simulink library "simetranss"  (R2024b)
settings: Solver=VariableStepAuto  StartTime=0.0  StopTime=10.0  RelTol=1e-3
PostLoadFcn:
  | Ts=1e-6
InitFcn:
  | Ts=1e-6
undefined symbols (not defined in the file): C, C_601, C_603, C_606, CC, Csnu, Csnubber, DiscIntNeverNeededParam, DPL, DPL1ph, FluxTable, ft2km, gcbh, h, Half, Imap2, L, L_601, L_603, L_606, Lbase, LpejoSw, Newton, R_601, R_603, R_606, Raphson, ResistanceM, Roff, Ron, RotorAngles, Rsnu, Rsnubber, Rt4, SampleTime, simetran, sps, sps_rtmsupport, StatorCurrents, T_2wind_ratio, T_Lpu, T_Lpu_pri, T_Rpu, T_Rpu_pri, T_Vpri, T_Vpri_15comp, T_Vsec, Ti, Ts_Power, Z, Zbase, Zm
libraries: fl_lib x248, ee_lib x146, nesl_utility x122, $bdroot x29, simulink x15, eeGeneralControl x2, spsStairGeneratorLib x2, artemis x1
(part 11 of 12)

== system simetranss/Passive/MATE Unbalanced LoadDEV1/RLseriesD ==
  Inductor : ee_lib/Passive/Inductor  l=L(1) H  enable_L_tol=ee.enum.toleranceApplication.none  L_tol=20  tol_distribution=ee.enum.toleranceDistribution.uniform  nSigma=4  r=0 Ohm  g=1e-9 1/Ohm  enable_operating_limits=ee.enum.enable.no  operating_limit_action=ee.enum.passive.reportOpLim.warn  max_working_current=1 A  power_rating=1 W  fault_action=simscape.enum.assert.action.none  t_fault=1 s  i_L_specify=off  i_L_priority=High  i_L=0 A  i_L_nominal_specify=off  i_L_nominal_value=1  i_L_nominal_unit=A
  Inductor1 : ee_lib/Passive/Inductor  l=L(2) H  enable_L_tol=ee.enum.toleranceApplication.none  L_tol=20  tol_distribution=ee.enum.toleranceDistribution.uniform  nSigma=4  r=0 Ohm  g=1e-9 1/Ohm  enable_operating_limits=ee.enum.enable.no  operating_limit_action=ee.enum.passive.reportOpLim.warn  max_working_current=1 A  power_rating=1 W  fault_action=simscape.enum.assert.action.none  t_fault=1 s  i_L_specify=off  i_L_priority=High  i_L=0 A  i_L_nominal_specify=off  i_L_nominal_value=1  i_L_nominal_unit=A
  Inductor2 : ee_lib/Passive/Inductor  l=L(3) H  enable_L_tol=ee.enum.toleranceApplication.none  L_tol=20  tol_distribution=ee.enum.toleranceDistribution.uniform  nSigma=4  r=0 Ohm  g=1e-9 1/Ohm  enable_operating_limits=ee.enum.enable.no  operating_limit_action=ee.enum.passive.reportOpLim.warn  max_working_current=1 A  power_rating=1 W  fault_action=simscape.enum.assert.action.none  t_fault=1 s  i_L_specify=off  i_L_priority=High  i_L=0 A  i_L_nominal_specify=off  i_L_nominal_value=1  i_L_nominal_unit=A
  Phase Splitter2 : ee_lib/Connectors & References/Phase Splitter
  Resistor : ee_lib/Passive/Resistor  R=R(1) Ohm  enable_R_tol=ee.enum.toleranceApplication.none  R_tol=5  tol_distribution=ee.enum.toleranceDistribution.uniform  nSigma=4  enable_operating_limits=ee.enum.enable.no  operating_limit_action=ee.enum.passive.reportOpLim.warn  power_rating=1 W  max_working_voltage=100 V  noise_mode=ee.enum.sources.noise.Disabled  Tdevice=25 degC  sample_time=1e-3 s  repeatability=ee.enum.ic.repeatability.notRepeatable  user_seed=0  auto_seed=1853927660  fault_action=simscape.enum.assert.action.none  t_fault=1 s  power_derating_T1=70 degC  power_derating_T2=155 degC  operating_temperature_range_vec=[-50, 150] degC  alpha=3.93e-3 1/K  Tmeas=25 degC  thermal_mass=100 J/K  temperature_specify=off  temperature_priority=High  temperature=298.15 K  temperature_nominal_specify=off  temperature_nominal_value=1  temperature_nominal_unit=K
  Resistor1 : ee_lib/Passive/Resistor  R=R(2) Ohm  enable_R_tol=ee.enum.toleranceApplication.none  R_tol=5  tol_distribution=ee.enum.toleranceDistribution.uniform  nSigma=4  enable_operating_limits=ee.enum.enable.no  operating_limit_action=ee.enum.passive.reportOpLim.warn  power_rating=1 W  max_working_voltage=100 V  noise_mode=ee.enum.sources.noise.Disabled  Tdevice=25 degC  sample_time=1e-3 s  repeatability=ee.enum.ic.repeatability.notRepeatable  user_seed=0  auto_seed=66516699  fault_action=simscape.enum.assert.action.none  t_fault=1 s  power_derating_T1=70 degC  power_derating_T2=155 degC  operating_temperature_range_vec=[-50, 150] degC  alpha=3.93e-3 1/K  Tmeas=25 degC  thermal_mass=100 J/K  temperature_specify=off  temperature_priority=High  temperature=298.15 K  temperature_nominal_specify=off  temperature_nominal_value=1  temperature_nominal_unit=K
  Resistor2 : ee_lib/Passive/Resistor  R=R(3) Ohm  enable_R_tol=ee.enum.toleranceApplication.none  R_tol=5  tol_distribution=ee.enum.toleranceDistribution.uniform  nSigma=4  enable_operating_limits=ee.enum.enable.no  operating_limit_action=ee.enum.passive.reportOpLim.warn  power_rating=1 W  max_working_voltage=100 V  noise_mode=ee.enum.sources.noise.Disabled  Tdevice=25 degC  sample_time=1e-3 s  repeatability=ee.enum.ic.repeatability.notRepeatable  user_seed=0  auto_seed=4226521513  fault_action=simscape.enum.assert.action.none  t_fault=1 s  power_derating_T1=70 degC  power_derating_T2=155 degC  operating_temperature_range_vec=[-50, 150] degC  alpha=3.93e-3 1/K  Tmeas=25 degC  thermal_mass=100 J/K  temperature_specify=off  temperature_priority=High  temperature=298.15 K  temperature_nominal_specify=off  temperature_nominal_value=1  temperature_nominal_unit=K
  Conn1 : PMIOPort  Side=Left
  connections:
  Inductor2/LConn1 -- Resistor2/RConn1
  Inductor/LConn1 -- Resistor/RConn1
  Inductor1/LConn1 -- Resistor1/RConn1
  Conn1/RConn1 -- Phase Splitter2/LConn1
  Phase Splitter2/RConn1 -- Inductor2/RConn1 -- Resistor/LConn1
  Inductor/RConn1 -- Resistor1/LConn1 -- Phase Splitter2/RConn2
  Inductor1/RConn1 -- Resistor2/LConn1 -- Phase Splitter2/RConn3

== system simetranss/Power converters/MATE_3LevelNPCinverter/Subsystem ==
  g : Inport
  Capacitor : fl_lib/Electrical/Electrical Elements/Capacitor  c=SnubberCapacitance F  r=0 Ohm  g=0 1/Ohm  i_specify=off  i_priority=None  i=0 A  i_nominal_specify=off  i_nominal_value=1  i_nominal_unit=A  v_specify=off  v_priority=None  v=0 V  v_nominal_specify=off  v_nominal_value=1  v_nominal_unit=V  vc_specify=off  vc_priority=High  vc=0 V  vc_nominal_specify=off  vc_nominal_value=1  vc_nominal_unit=V
  Resistor : fl_lib/Electrical/Electrical Elements/Resistor  R=SnubberResistance Ohm  i_specify=off  i_priority=None  i=0 A  i_nominal_specify=off  i_nominal_value=1  i_nominal_unit=A  v_specify=off  v_priority=None  v=0 V  v_nominal_specify=off  v_nominal_value=1  v_nominal_unit=V
  SPST Switch : ee_lib/Switches & Breakers/SPST Switch  R_closed=Ron*2 Ohm  G_open=1e-6 S  Threshold=0.5 V  Width=0 V  model_dynamics=0  t_on=1e-3 s  t_off=1e-3 s  initial_vT=0 V
      settings: InternalSimscapePortConfiguration="{\"Bottom\":[],\"Left\":[{\"id\":\"vT\",\"label\":\"vT\",\"type\":\"input\"},{\"id\":\"p\",\"label\":\"\",\"type\":\"foundation.electrical.electrical\"}],\"Right\":[{\"id\":\"n\",\"label\":\"\",\"type\":\"foundation.electrical.electrical\"}],\"Top\":[]}"
  Simulink-PS Converter : nesl_utility/Simulink-PS Converter  PhysicalDomain=network_engine_domain  SubClassName=ps_input  LeftPortType=input  RightPortType=output  PseudoPeriodic=off  Frequencies=[]  NoiseDistribution=none  NoiseParameters=[]  Unit=1  AffineConversion=off  FilteringAndDerivatives=provide  SimscapeFilterOrder=1  InputFilterTimeConstant=0.001  UdotUserProvided=0
  P : PMIOPort  Side=Left
  N : PMIOPort  Port=2  Side=Right
  wires:
  g/1 -> Simulink-PS Converter/1
  connections:
  SPST Switch/LConn2 -- Capacitor/LConn1 -- P/RConn1
  Simulink-PS Converter/RConn1 -- SPST Switch/LConn1
  SPST Switch/RConn1 -- Resistor/RConn1 -- N/RConn1
  Capacitor/RConn1 -- Resistor/LConn1

== system simetranss/Power converters/MATE_3LevelNPCinverter/Subsystem1 ==
  g : Inport
  Capacitor : fl_lib/Electrical/Electrical Elements/Capacitor  c=SnubberCapacitance F  r=0 Ohm  g=0 1/Ohm  i_specify=off  i_priority=None  i=0 A  i_nominal_specify=off  i_nominal_value=1  i_nominal_unit=A  v_specify=off  v_priority=None  v=0 V  v_nominal_specify=off  v_nominal_value=1  v_nominal_unit=V  vc_specify=off  vc_priority=High  vc=0 V  vc_nominal_specify=off  vc_nominal_value=1  vc_nominal_unit=V
  Resistor : fl_lib/Electrical/Electrical Elements/Resistor  R=SnubberResistance Ohm  i_specify=off  i_priority=None  i=0 A  i_nominal_specify=off  i_nominal_value=1  i_nominal_unit=A  v_specify=off  v_priority=None  v=0 V  v_nominal_specify=off  v_nominal_value=1  v_nominal_unit=V
  SPST Switch : ee_lib/Switches & Breakers/SPST Switch  R_closed=Ron*2 Ohm  G_open=1e-6 S  Threshold=0.5 V  Width=0 V  model_dynamics=0  t_on=1e-3 s  t_off=1e-3 s  initial_vT=0 V
      settings: InternalSimscapePortConfiguration="{\"Bottom\":[],\"Left\":[{\"id\":\"vT\",\"label\":\"vT\",\"type\":\"input\"},{\"id\":\"p\",\"label\":\"\",\"type\":\"foundation.electrical.electrical\"}],\"Right\":[{\"id\":\"n\",\"label\":\"\",\"type\":\"foundation.electrical.electrical\"}],\"Top\":[]}"
  Simulink-PS Converter : nesl_utility/Simulink-PS Converter  PhysicalDomain=network_engine_domain  SubClassName=ps_input  LeftPortType=input  RightPortType=output  PseudoPeriodic=off  Frequencies=[]  NoiseDistribution=none  NoiseParameters=[]  Unit=1  AffineConversion=off  FilteringAndDerivatives=provide  SimscapeFilterOrder=1  InputFilterTimeConstant=0.001  UdotUserProvided=0
  P : PMIOPort  Side=Left
  N : PMIOPort  Port=2  Side=Right
  wires:
  g/1 -> Simulink-PS Converter/1
  connections:
  SPST Switch/LConn2 -- Capacitor/LConn1 -- P/RConn1
  Simulink-PS Converter/RConn1 -- SPST Switch/LConn1
  SPST Switch/RConn1 -- Resistor/RConn1 -- N/RConn1
  Capacitor/RConn1 -- Resistor/LConn1

== system simetranss/Power converters/MATE_3LevelNPCinverter/Subsystem2 ==
  g : Inport
  Capacitor : fl_lib/Electrical/Electrical Elements/Capacitor  c=SnubberCapacitance F  r=0 Ohm  g=0 1/Ohm  i_specify=off  i_priority=None  i=0 A  i_nominal_specify=off  i_nominal_value=1  i_nominal_unit=A  v_specify=off  v_priority=None  v=0 V  v_nominal_specify=off  v_nominal_value=1  v_nominal_unit=V  vc_specify=off  vc_priority=High  vc=0 V  vc_nominal_specify=off  vc_nominal_value=1  vc_nominal_unit=V
  Resistor : fl_lib/Electrical/Electrical Elements/Resistor  R=SnubberResistance Ohm  i_specify=off  i_priority=None  i=0 A  i_nominal_specify=off  i_nominal_value=1  i_nominal_unit=A  v_specify=off  v_priority=None  v=0 V  v_nominal_specify=off  v_nominal_value=1  v_nominal_unit=V
  SPST Switch : ee_lib/Switches & Breakers/SPST Switch  R_closed=Ron*2 Ohm  G_open=1e-6 S  Threshold=0.5 V  Width=0 V  model_dynamics=0  t_on=1e-3 s  t_off=1e-3 s  initial_vT=0 V
      settings: InternalSimscapePortConfiguration="{\"Bottom\":[],\"Left\":[{\"id\":\"vT\",\"label\":\"vT\",\"type\":\"input\"},{\"id\":\"p\",\"label\":\"\",\"type\":\"foundation.electrical.electrical\"}],\"Right\":[{\"id\":\"n\",\"label\":\"\",\"type\":\"foundation.electrical.electrical\"}],\"Top\":[]}"
  Simulink-PS Converter : nesl_utility/Simulink-PS Converter  PhysicalDomain=network_engine_domain  SubClassName=ps_input  LeftPortType=input  RightPortType=output  PseudoPeriodic=off  Frequencies=[]  NoiseDistribution=none  NoiseParameters=[]  Unit=1  AffineConversion=off  FilteringAndDerivatives=provide  SimscapeFilterOrder=1  InputFilterTimeConstant=0.001  UdotUserProvided=0
  P : PMIOPort  Side=Left
  N : PMIOPort  Port=2  Side=Right
  wires:
  g/1 -> Simulink-PS Converter/1
  connections:
  Capacitor/RConn1 -- Resistor/LConn1
  N/RConn1 -- Resistor/RConn1 -- SPST Switch/RConn1
  Simulink-PS Converter/RConn1 -- SPST Switch/LConn1
  P/RConn1 -- Capacitor/LConn1 -- SPST Switch/LConn2

== system simetranss/Power converters/MATE_MMCarm/Subsystem ==
  gup : Inport
  en : Inport  Port=2
  Compare To Constant : simulink/Logic and Bit Operations/Compare To Constant  relop=>=  const=0.5  OutDataTypeStr=boolean
  Data Type Conversion : DataTypeConversion  OutDataTypeStr=double  SaturateOnIntegerOverflow=off  RndMeth=Floor
  Data Type Conversion1 : DataTypeConversion  OutDataTypeStr=double  SaturateOnIntegerOverflow=off  RndMeth=Floor
  Divide : Product
  Divide1 : Product
  Logical Operator1 : Logic  Operator=NOT  Inputs=1  AllPortsSameDT=off  OutDataTypeStr=boolean
  out : Outport  VectorParamsAs1DForOutWhenUnconnected=off
  outN : Outport  Port=2  VectorParamsAs1DForOutWhenUnconnected=off
  wires:
  gup/1 -> Compare To Constant/1
  Logical Operator1/1 -> Data Type Conversion/1
  Compare To Constant/1 -> Data Type Conversion1/1, Logical Operator1/1
  en/1 -> Divide/1, Divide1/2
  Data Type Conversion/1 -> Divide1/1
  Data Type Conversion1/1 -> Divide/2
  Divide/1 -> out/1
  Divide1/1 -> outN/1

== system simetranss/Power converters/Switching Function Interpolating 2-level inverter/ctrl1 ==
  g : Inport
  g1 : Inport  Port=2
  Iac : Inport  Port=3
  Vdc : Inport  Port=4
  Compare To Zero : simulink/Logic and Bit Operations/Compare To Zero  relop=>  OutDataTypeStr=uint8
  Constant : Constant
  Constant1 : Constant  Value=0
  Data Type Conversion1 : DataTypeConversion  OutDataTypeStr=double  SaturateOnIntegerOverflow=off  RndMeth=Floor
  Divide : Product  Inputs=3
  Divide1 : Product
  Divide3 : Product
  Logical Operator7 : Logic  Operator=NOT  AllPortsSameDT=off  OutDataTypeStr=boolean
  Relational Operator2 : RelationalOperator  Operator=~=  OutDataTypeStr=boolean  InputSameDT=off
  Sum : Sum  Inputs=|++
  Sum1 : Sum  Inputs=--+
  Sum2 : Sum  Inputs=|++
  Idc : Outport  VectorParamsAs1DForOutWhenUnconnected=off
  Vac : Outport  Port=2  VectorParamsAs1DForOutWhenUnconnected=off
  sw : Outport  Port=3  VectorParamsAs1DForOutWhenUnconnected=off
  wires:
  Divide3/1 -> Sum2/2
  Sum1/1 -> Divide3/2
  Constant/1 -> Sum1/3
  Logical Operator7/1 -> Divide3/1
  g1/1 -> Sum1/2, Sum/2
  Data Type Conversion1/1 -> sw/1, Divide/3
  Vdc/1 -> Divide1/1
  Compare To Zero/1 -> Logical Operator7/1
  g/1 -> Sum1/1, Sum/1, Sum2/1
  Sum2/1 -> Divide1/2, Divide/2
  Divide1/1 -> Vac/1
  Divide/1 -> Idc/1
  Iac/1 -> Compare To Zero/1, Divide/1
  Sum/1 -> Relational Operator2/1
  Constant1/1 -> Relational Operator2/2
  Relational Operator2/1 -> Data Type Conversion1/1

== system simetranss/Power converters/Switching Function Interpolating 2-level inverter/lowthy ==
  g : Inport
  i : Inport  Port=2
  Capacitor : fl_lib/Electrical/Electrical Elements/Capacitor  c=Gi F  r=Gp Ohm  g=0 1/Ohm  i_specify=off  i_priority=None  i=0 A  i_nominal_specify=off  i_nominal_value=1  i_nominal_unit=A  v_specify=off  v_priority=None  v=0 V  v_nominal_specify=off  v_nominal_value=1  v_nominal_unit=V  vc_specify=off  vc_priority=High  vc=0 V  vc_nominal_specify=off  vc_nominal_value=1  vc_nominal_unit=V
  Compare To Zero : simulink/Logic and Bit Operations/Compare To Zero  relop=<  OutDataTypeStr=boolean
  Compare To Zero1 : simulink/Logic and Bit Operations/Compare To Zero  relop=>  OutDataTypeStr=boolean
  Data Type Conversion1 : DataTypeConversion  OutDataTypeStr=double  SaturateOnIntegerOverflow=off  RndMeth=Floor
  Logical Operator1 : Logic  Operator=OR  Inputs=3  AllPortsSameDT=off  OutDataTypeStr=boolean
  Logical Operator10 : Logic  Operator=NOT  Inputs=1  AllPortsSameDT=off  OutDataTypeStr=boolean
  Logical Operator11 : Logic  Inputs=3  AllPortsSameDT=off  OutDataTypeStr=boolean
  Logical Operator{2..4,7} (4 alike) : Logic  AllPortsSameDT=off  OutDataTypeStr=boolean
  Logical Operator5 : Logic  Operator=NOT  Inputs=1  AllPortsSameDT=off  OutDataTypeStr=boolean
  Logical Operator6 : Logic  Operator=OR  AllPortsSameDT=off  OutDataTypeStr=boolean
  Mem{1..5} (5 alike) : Memory  InheritSampleTime=on
  PS-Simulink Converter1 : nesl_utility/PS-Simulink Converter  PhysicalDomain=network_engine_domain  SubClassName=ps_output  LeftPortType=input  RightPortType=output  PseudoPeriodic=off  Frequencies=[]  VectorFormat=inherit  Unit=inherit  AffineConversion=off
  Simulink-PS Converter3 : nesl_utility/Simulink-PS Converter  PhysicalDomain=network_engine_domain  SubClassName=ps_input  LeftPortType=input  RightPortType=output  PseudoPeriodic=off  Frequencies=[]  NoiseDistribution=none  NoiseParameters=[]  Unit=1  AffineConversion=off  FilteringAndDerivatives=provide  SimscapeFilterOrder=1  InputFilterTimeConstant=0.001  UdotUserProvided=0
  Switch : fl_lib/Electrical/Electrical Elements/Switch  R_closed=Ron Ohm  G_open=1e-8 1/Ohm  Threshold=0.5  i_specify=off  i_priority=None  i=0 A  i_nominal_specify=off  i_nominal_value=1  i_nominal_unit=A  v_specify=off  v_priority=None  v=0 V  v_nominal_specify=off  v_nominal_value=1  v_nominal_unit=V
  Voltage Sensor1 : fl_lib/Electrical/Electrical Sensors/Voltage Sensor
  + : PMIOPort  Side=Right
  - : PMIOPort  Port=2  Side=Left
  wires:
  Data Type Conversion1/1 -> Simulink-PS Converter3/1
  PS-Simulink Converter1/1 -> Mem1/1
  Logical Operator3/1 -> Data Type Conversion1/1
  Mem4/1 -> Logical Operator11/1
  Compare To Zero1/1 -> Logical Operator11/3
  g/1 -> Logical Operator4/2, Logical Operator11/2, Logical Operator10/1
  Mem5/1 -> Compare To Zero1/1
  Mem2/1 -> Logical Operator2/2
  Logical Operator2/1 -> Logical Operator1/1
  Logical Operator4/1 -> Logical Operator1/2
  Logical Operator1/1 -> Logical Operator7/1, Logical Operator3/1
  Mem1/1 -> Compare To Zero/1
  Compare To Zero/1 -> Logical Operator4/1, Logical Operator2/1
  Logical Operator10/1 -> Mem4/1, Logical Operator5/1, Mem3/1
  Mem3/1 -> Logical Operator6/1
  Logical Operator5/1 -> Logical Operator6/2
  Logical Operator6/1 -> Logical Operator3/2, Logical Operator7/2
  i/1 -> Mem5/1
  Logical Operator11/1 -> Logical Operator1/3
  Logical Operator7/1 -> Mem2/1
  connections:
  PS-Simulink Converter1/LConn1 -- Voltage Sensor1/RConn1
  Simulink-PS Converter3/RConn1 -- Switch/RConn1
  +/RConn1 -- Capacitor/LConn1 -- Voltage Sensor1/LConn1 -- Switch/RConn2
  -/RConn1 -- Capacitor/RConn1 -- Voltage Sensor1/RConn2 -- Switch/LConn1

== system simetranss/Power converters/Switching Function Interpolating 2-level inverter/upthy ==
  g : Inport
  "i " : Inport  Port=2
  Capacitor : fl_lib/Electrical/Electrical Elements/Capacitor  c=Gi F  r=Gp Ohm  g=0 1/Ohm  i_specify=off  i_priority=None  i=0 A  i_nominal_specify=off  i_nominal_value=1  i_nominal_unit=A  v_specify=off  v_priority=None  v=0 V  v_nominal_specify=off  v_nominal_value=1  v_nominal_unit=V  vc_specify=off  vc_priority=High  vc=0 V  vc_nominal_specify=off  vc_nominal_value=1  vc_nominal_unit=V
  Compare To Zero : simulink/Logic and Bit Operations/Compare To Zero  relop=<  OutDataTypeStr=boolean
  Compare To Zero2 : simulink/Logic and Bit Operations/Compare To Zero  relop=<  OutDataTypeStr=boolean
  Data Type Conversion1 : DataTypeConversion  OutDataTypeStr=double  SaturateOnIntegerOverflow=off  RndMeth=Floor
  Logical Operator1 : Logic  Operator=OR  Inputs=3  AllPortsSameDT=off  OutDataTypeStr=boolean
  Logical Operator10 : Logic  Operator=NOT  Inputs=1  AllPortsSameDT=off  OutDataTypeStr=boolean
  Logical Operator11 : Logic  Inputs=3  AllPortsSameDT=off  OutDataTypeStr=boolean
  Logical Operator{2..4,7} (4 alike) : Logic  AllPortsSameDT=off  OutDataTypeStr=boolean
  Logical Operator5 : Logic  Operator=NOT  Inputs=1  AllPortsSameDT=off  OutDataTypeStr=boolean
  Logical Operator6 : Logic  Operator=OR  AllPortsSameDT=off  OutDataTypeStr=boolean
  Mem{1..3,6..7} (5 alike) : Memory  InheritSampleTime=on
  PS-Simulink Converter1 : nesl_utility/PS-Simulink Converter  PhysicalDomain=network_engine_domain  SubClassName=ps_output  LeftPortType=input  RightPortType=output  PseudoPeriodic=off  Frequencies=[]  VectorFormat=inherit  Unit=inherit  AffineConversion=off
  Simulink-PS Converter3 : nesl_utility/Simulink-PS Converter  PhysicalDomain=network_engine_domain  SubClassName=ps_input  LeftPortType=input  RightPortType=output  PseudoPeriodic=off  Frequencies=[]  NoiseDistribution=none  NoiseParameters=[]  Unit=1  AffineConversion=off  FilteringAndDerivatives=provide  SimscapeFilterOrder=1  InputFilterTimeConstant=0.001  UdotUserProvided=0
  Switch : fl_lib/Electrical/Electrical Elements/Switch  R_closed=Ron Ohm  G_open=1e-8 1/Ohm  Threshold=0.5  i_specify=off  i_priority=None  i=0 A  i_nominal_specify=off  i_nominal_value=1  i_nominal_unit=A  v_specify=off  v_priority=None  v=0 V  v_nominal_specify=off  v_nominal_value=1  v_nominal_unit=V
  Voltage Sensor1 : fl_lib/Electrical/Electrical Sensors/Voltage Sensor
  + : PMIOPort  Side=Right
  - : PMIOPort  Port=2  Side=Left
  wires:
  Data Type Conversion1/1 -> Simulink-PS Converter3/1
  Mem2/1 -> Logical Operator2/2
  Logical Operator2/1 -> Logical Operator1/1
  Logical Operator4/1 -> Logical Operator1/2
  Logical Operator1/1 -> Logical Operator7/1, Logical Operator3/1
  Mem1/1 -> Compare To Zero/1
  PS-Simulink Converter1/1 -> Mem1/1
  Compare To Zero/1 -> Logical Operator4/1, Logical Operator2/1
  Logical Operator3/1 -> Data Type Conversion1/1
  Logical Operator10/1 -> Mem6/1, Mem3/1, Logical Operator5/1
  Mem3/1 -> Logical Operator6/1
  Logical Operator5/1 -> Logical Operator6/2
  Logical Operator6/1 -> Logical Operator3/2, Logical Operator7/2
  "i "/1 -> Mem7/1
  Mem7/1 -> Compare To Zero2/1
  g/1 -> Logical Operator4/2, Logical Operator10/1, Logical Operator11/1
  Mem6/1 -> Logical Operator11/2
  Compare To Zero2/1 -> Logical Operator11/3
  Logical Operator11/1 -> Logical Operator1/3
  Logical Operator7/1 -> Mem2/1
  connections:
  Simulink-PS Converter3/RConn1 -- Switch/RConn1
  Voltage Sensor1/RConn1 -- PS-Simulink Converter1/LConn1
  Capacitor/RConn1 -- -/RConn1 -- Switch/LConn1 -- Voltage Sensor1/RConn2
  Capacitor/LConn1 -- +/RConn1 -- Switch/RConn2 -- Voltage Sensor1/LConn1

== system simetranss/Switches/MATE 3ph Breaker/RCsnubber ==
  Capacitor : ee_lib/Passive/Capacitor  cap_option=ee.enum.passive.capacitor.capOption.const  c=SnubberCapacitance F  Cvec=[1e-05, 1e-06] F  Vvec=[0, 10] V  CV_table_symmetry=ee.enum.passive.capacitor.tableSymmetry.yes  f_vec=[1, 10] kHz  DFext_vec=[.8, 1.2]  enable_C_tol=ee.enum.toleranceApplication.none  averaging_period=0 s  C_tol=5  tol_distribution=ee.enum.toleranceDistribution.uniform  nSigma=4  r=SnubberResistance Ohm  g=0 1/Ohm  enable_operating_limits=ee.enum.enable.no  operating_limit_action=ee.enum.passive.reportOpLim.warn  max_working_voltage_range=[-25, 25] V  power_rating=1 W  maxTemperature=85 degC  thermalEnable=false  thermalMass=1 J/K  fault_action=simscape.enum.assert.action.none  t_fault=1 s  i_specify=off  i_priority=None  i=0 A  i_nominal_specify=off  i_nominal_value=1  i_nominal_unit=A  v_specify=off  v_priority=None  v=0 V  v_nominal_specify=off  v_nominal_value=1  v_nominal_unit=V  vc_specify=off  vc_priority=High  vc=0 V  vc_nominal_specify=off  vc_nominal_value=1  vc_nominal_unit=V  T_specify=off  T_priority=None  T=298.15 K  T_nominal_specify=off  T_nominal_value=1  T_nominal_unit=K
  Capacitor1 : ee_lib/Passive/Capacitor  cap_option=ee.enum.passive.capacitor.capOption.const  c=SnubberCapacitance F  Cvec=[1e-05, 1e-06] F  Vvec=[0, 10] V  CV_table_symmetry=ee.enum.passive.capacitor.tableSymmetry.yes  f_vec=[1, 10] kHz  DFext_vec=[.8, 1.2]  enable_C_tol=ee.enum.toleranceApplication.none  averaging_period=0 s  C_tol=5  tol_distribution=ee.enum.toleranceDistribution.uniform  nSigma=4  r=SnubberResistance Ohm  g=0 1/Ohm  enable_operating_limits=ee.enum.enable.no  operating_limit_action=ee.enum.passive.reportOpLim.warn  max_working_voltage_range=[-25, 25] V  power_rating=1 W  maxTemperature=85 degC  thermalEnable=false  thermalMass=1 J/K  fault_action=simscape.enum.assert.action.none  t_fault=1 s  i_specify=off  i_priority=None  i=0 A  i_nominal_specify=off  i_nominal_value=1  i_nominal_unit=A  v_specify=off  v_priority=None  v=0 V  v_nominal_specify=off  v_nominal_value=1  v_nominal_unit=V  vc_specify=off  vc_priority=High  vc=0 V  vc_nominal_specify=off  vc_nominal_value=1  vc_nominal_unit=V  T_specify=off  T_priority=None  T=298.15 K  T_nominal_specify=off  T_nominal_value=1  T_nominal_unit=K
  Capacitor2 : ee_lib/Passive/Capacitor  cap_option=ee.enum.passive.capacitor.capOption.const  c=SnubberCapacitance F  Cvec=[1e-05, 1e-06] F  Vvec=[0, 10] V  CV_table_symmetry=ee.enum.passive.capacitor.tableSymmetry.yes  f_vec=[1, 10] kHz  DFext_vec=[.8, 1.2]  enable_C_tol=ee.enum.toleranceApplication.none  averaging_period=0 s  C_tol=5  tol_distribution=ee.enum.toleranceDistribution.uniform  nSigma=4  r=SnubberResistance Ohm  g=0 1/Ohm  enable_operating_limits=ee.enum.enable.no  operating_limit_action=ee.enum.passive.reportOpLim.warn  max_working_voltage_range=[-25, 25] V  power_rating=1 W  maxTemperature=85 degC  thermalEnable=false  thermalMass=1 J/K  fault_action=simscape.enum.assert.action.none  t_fault=1 s  i_specify=off  i_priority=None  i=0 A  i_nominal_specify=off  i_nominal_value=1  i_nominal_unit=A  v_specify=off  v_priority=None  v=0 V  v_nominal_specify=off  v_nominal_value=1  v_nominal_unit=V  vc_specify=off  vc_priority=High  vc=0 V  vc_nominal_specify=off  vc_nominal_value=1  vc_nominal_unit=V  T_specify=off  T_priority=None  T=298.15 K  T_nominal_specify=off  T_nominal_value=1  T_nominal_unit=K
  Conn1 : PMIOPort  Side=Left
  Conn2 : PMIOPort  Port=2  Side=Left
  Conn3 : PMIOPort  Port=3  Side=Left
  Conn4 : PMIOPort  Port=4  Side=Right
  Conn5 : PMIOPort  Port=5  Side=Right
  Conn6 : PMIOPort  Port=6  Side=Right
  connections:
  Conn4/RConn1 -- Capacitor/RConn1
  Conn6/RConn1 -- Capacitor2/RConn1
  Conn2/RConn1 -- Capacitor1/LConn1
  Capacitor/LConn1 -- Conn3/RConn1
  Conn1/RConn1 -- Capacitor2/LConn1
  Conn5/RConn1 -- Capacitor1/RConn1

== system simetranss/Switches/MATE Breaker/RCsnubber ==
  Capacitor2 : ee_lib/Passive/Capacitor  cap_option=ee.enum.passive.capacitor.capOption.const  c=SnubberCapacitance F  Cvec=[1e-05, 1e-06] F  Vvec=[0, 10] V  CV_table_symmetry=ee.enum.passive.capacitor.tableSymmetry.yes  f_vec=[1, 10] kHz  DFext_vec=[.8, 1.2]  enable_C_tol=ee.enum.toleranceApplication.none  averaging_period=0 s  C_tol=5  tol_distribution=ee.enum.toleranceDistribution.uniform  nSigma=4  r=SnubberResistance Ohm  g=0 1/Ohm  enable_operating_limits=ee.enum.enable.no  operating_limit_action=ee.enum.passive.reportOpLim.warn  max_working_voltage_range=[-25, 25] V  power_rating=1 W  maxTemperature=85 degC  thermalEnable=false  thermalMass=1 J/K  fault_action=simscape.enum.assert.action.none  t_fault=1 s  i_specify=off  i_priority=None  i=0 A  i_nominal_specify=off  i_nominal_value=1  i_nominal_unit=A  v_specify=off  v_priority=None  v=0 V  v_nominal_specify=off  v_nominal_value=1  v_nominal_unit=V  vc_specify=off  vc_priority=High  vc=0 V  vc_nominal_specify=off  vc_nominal_value=1  vc_nominal_unit=V  T_specify=off  T_priority=None  T=298.15 K  T_nominal_specify=off  T_nominal_value=1  T_nominal_unit=K
  Conn1 : PMIOPort  Side=Left
  Conn6 : PMIOPort  Port=2  Side=Right
  connections:
  Conn1/RConn1 -- Capacitor2/LConn1
  Conn6/RConn1 -- Capacitor2/RConn1

== system simetranss/FPGA/MATE 2level_Inverter SwitchingFunction(3ph)/SW/INT ==
  u : Inport
  Initial : Inport  Port=2
  en : Inport  Port=3
  Gain1 : Gain  Gain=-Ts/Gi
  Logical Operator10 : Logic  Operator=NOT  AllPortsSameDT=off  OutDataTypeStr=boolean
  Saturation : Saturate  UpperLimit=inf  LowerLimit=0
  Sum : Sum  Inputs=|++
  Switch1 : Switch  Criteria=u2 ~= 0  SaturateOnIntegerOverflow=off  InputSameDT=off
  Unit Delay1 : UnitDelay  SampleTime=Ts  HasFrameUpgradeWarning=on
  u_p : Outport  VectorParamsAs1DForOutWhenUnconnected=off
  wires:
  Gain1/1 -> Sum/1
  en/1 -> Logical Operator10/1
  Saturation/1 -> u_p/1, Unit Delay1/1
  Switch1/1 -> Sum/2
  u/1 -> Gain1/1
  Sum/1 -> Saturation/1
  Unit Delay1/1 -> Switch1/3
  Initial/1 -> Switch1/1
  Logical Operator10/1 -> Switch1/2

== system simetranss/FPGA/MATE 2level_InverterSWHIZ/SW/INT ==
  u : Inport
  Initial : Inport  Port=2
  en : Inport  Port=3
  Logical Operator10 : Logic  Operator=NOT  AllPortsSameDT=off  OutDataTypeStr=boolean
  Saturation : Saturate  Commented=through  UpperLimit=inf  LowerLimit=0
  Sum : Sum  Inputs=|-+
  Switch1 : Switch  Criteria=u2 ~= 0  SaturateOnIntegerOverflow=off  InputSameDT=off
  Unit Delay1 : UnitDelay  SampleTime=Ts  HasFrameUpgradeWarning=on
  u_p : Outport  VectorParamsAs1DForOutWhenUnconnected=off
  wires:
  u/1 -> Sum/1
  en/1 -> Logical Operator10/1
  Saturation/1 -> u_p/1, Unit Delay1/1
  Switch1/1 -> Sum/2
  Sum/1 -> Saturation/1
  Unit Delay1/1 -> Switch1/3
  Initial/1 -> Switch1/1
  Logical Operator10/1 -> Switch1/2

== system simetranss/FPGA/MATE 3levelNPC_Inverter SwitchingFunction(3ph)/SW/INT ==
  u : Inport
  Initial : Inport  Port=2
  en : Inport  Port=3
  Gain1 : Gain  Gain=-Ts/Gi
  Logical Operator10 : Logic  Operator=NOT  AllPortsSameDT=off  OutDataTypeStr=boolean
  Saturation : Saturate  UpperLimit=inf  LowerLimit=0
  Sum : Sum  Inputs=|++
  Switch1 : Switch  Criteria=u2 ~= 0  SaturateOnIntegerOverflow=off  InputSameDT=off
  Unit Delay1 : UnitDelay  SampleTime=Ts  HasFrameUpgradeWarning=on
  u_p : Outport  VectorParamsAs1DForOutWhenUnconnected=off
  wires:
  Unit Delay1/1 -> Switch1/3
  Gain1/1 -> Sum/1
  en/1 -> Logical Operator10/1
  Saturation/1 -> Unit Delay1/1, u_p/1
  Switch1/1 -> Sum/2
  u/1 -> Gain1/1
  Sum/1 -> Saturation/1
  Initial/1 -> Switch1/1
  Logical Operator10/1 -> Switch1/2

== system simetranss/FPGA/MATE 3levelNPC_Inverter SwitchingFunction(3ph)/SW/logic ==
  In1 : Inport
  In2 : Inport  Port=2
  Logical Operator4 : Logic  AllPortsSameDT=off  OutDataTypeStr=boolean
  Logical Operator5 : Logic  AllPortsSameDT=off  OutDataTypeStr=boolean
  Logical Operator6 : Logic  Operator=OR  Inputs=3  AllPortsSameDT=off  OutDataTypeStr=boolean
  Logical Operator8 : Logic  AllPortsSameDT=off  OutDataTypeStr=boolean
  Logical Operator9 : Logic  Operator=NOT  AllPortsSameDT=off  OutDataTypeStr=boolean
  Unit Delay2 : UnitDelay  SampleTime=Ts  HasFrameUpgradeWarning=on
  Out1 : Outport
  wires:
  Logical Operator5/1 -> Logical Operator6/3
  In1/1 -> Logical Operator5/1, Logical Operator4/1
  Unit Delay2/1 -> Logical Operator9/1, Logical Operator8/2
  Logical Operator8/1 -> Logical Operator6/2
  Logical Operator9/1 -> Logical Operator4/2
  Logical Operator6/1 -> Unit Delay2/1, Out1/1
  Logical Operator4/1 -> Logical Operator6/1
  In2/1 -> Logical Operator8/1, Logical Operator5/2

== system simetranss/Lines/Half-DPL/dplmodel/Subsystem ==
  In1 : Inport
  Add : Sum
  Delay : Delay  DelayLength=delay(2)
  Delay1 : Delay  DelayLength=delay(1)
  Delay2 : Delay  DelayLength=delay(2)
  Demux : Demux  Outputs=3
  Gain : Gain  Gain=remd
  Gain1 : Gain  Gain=1-remd
  Mux : Mux  Inputs=3
  Mux1 : Mux  Inputs=3
  Unit Delay : UnitDelay  SampleTime=Ts  HasFrameUpgradeWarning=on
  Unit Delay1 : UnitDelay  SampleTime=Ts  HasFrameUpgradeWarning=on
  Unit Delay2 : UnitDelay  SampleTime=Ts  HasFrameUpgradeWarning=on
  Out1 : Outport
  wires:
  In1/1 -> Demux/1
  Demux/2 -> Delay/1
  Demux/3 -> Delay2/1
  Demux/1 -> Delay1/1
  Delay1/1 -> Mux1/1, Unit Delay1/1
  Delay/1 -> Mux1/2, Unit Delay/1
  Delay2/1 -> Mux1/3, Unit Delay2/1
  Gain/1 -> Add/1
  Gain1/1 -> Add/2
  Unit Delay/1 -> Mux/2
  Unit Delay1/1 -> Mux/1
  Unit Delay2/1 -> Mux/3
  Add/1 -> Out1/1
  Mux/1 -> Gain/1
  Mux1/1 -> Gain1/1

== system simetranss/Lines/Half-DPL1ph/dplmodel/derlay ==
  In1 : Inport
  Add : Sum
  Delay1 : Delay  DelayLength=delay(1)
  Gain : Gain  Gain=remd
  Gain1 : Gain  Gain=1-remd
  Unit Delay1 : UnitDelay  SampleTime=Ts  HasFrameUpgradeWarning=on
  Out1 : Outport
  wires:
  In1/1 -> Delay1/1
  Gain/1 -> Add/1
  Gain1/1 -> Add/2
  Unit Delay1/1 -> Gain/1
  Add/1 -> Out1/1
  Delay1/1 -> Gain1/1, Unit Delay1/1

== system simetranss/Machines/MATE Synchronous Machine/Delta angle/Cartesian to Polar ==
  x : Inport
  y : Inport  Port=2
  Mux : Mux  Inputs=2
  x->r : Fcn  Expr=hypot(u[1],u[2])
  x->theta : Fcn  Expr=atan2(u[2],u[1])
  r : Outport  InitialOutput=0
  theta : Outport  Port=2  InitialOutput=0
  wires:
  x->theta/1 -> theta/1
  y/1 -> Mux/2
  x/1 -> Mux/1
  x->r/1 -> r/1
  Mux/1 -> x->r/1, x->theta/1

== system simetranss/Machines/MATE Synchronous Machine/Delta angle/Radians to Degrees ==
  Radians in : Inport
  Gain : Gain  Gain=180/pi  SaturateOnIntegerOverflow=on  OutDataTypeStr=Inherit: Same as input  ParamDataTypeStr=Inherit: Same as input
  Degrees out : Outport  InitialOutput=0
  wires:
  Radians in/1 -> Gain/1
  Gain/1 -> Degrees out/1

== system simetranss/Machines/MATE Synchronous Machine/SSS-SM equations/Discretize ==
  Ac : Inport
  Bc : Inport  Port=2
  Unity : Inport  Port=3
  Product1 : Product  Multiplication=Matrix(*)  SaturateOnIntegerOverflow=on  OutDataTypeStr=Inherit: Same as first input
  Product2 : Product  Multiplication=Matrix(*)  SaturateOnIntegerOverflow=on  OutDataTypeStr=Inherit: Same as first input
  Product4 : Product  Multiplication=Matrix(*)  SaturateOnIntegerOverflow=on  OutDataTypeStr=Inherit: Same as first input
  Sum1 : Sum  Inputs=+-  SaturateOnIntegerOverflow=on
  Sum5 : Sum  SaturateOnIntegerOverflow=on
  Ts/2 : Gain  Gain=Ts/2  SaturateOnIntegerOverflow=on  OutDataTypeStr=Inherit: Same as input  ParamDataTypeStr=Inherit: Same as input
  inversion : Product  Inputs=/  Multiplication=Matrix(*)  RndMeth=Zero
  trapeze has Ts/2 factor on B : Gain  Gain=Ts/2  SaturateOnIntegerOverflow=on  OutDataTypeStr=Inherit: Same as input  ParamDataTypeStr=Inherit: Same as input
  trapeze has Ts/2 factor on B1 : Gain  Gain=Ts/2  SaturateOnIntegerOverflow=on  OutDataTypeStr=Inherit: Same as input  ParamDataTypeStr=Inherit: Same as input
  Ad : Outport
  Bd : Outport  Port=2
  Bdin : Outport  Port=3
  wires:
  trapeze has Ts/2 factor on B1/1 -> Product2/2
  Product2/1 -> Bdin/1
  inversion/1 -> Product2/1, Product1/1, Product4/1  "inv(I4-Ts/2*A)"
  Bc/1 -> trapeze has Ts/2 factor on B/1
  trapeze has Ts/2 factor on B/1 -> Product1/2
  Ts/2/1 -> Sum5/2, Sum1/2
  Product4/1 -> Ad/1
  Unity/1 -> trapeze has Ts/2 factor on B1/1, Sum5/1, Sum1/1
  Sum5/1 -> Product4/2
  Product1/1 -> Bd/1
  Ac/1 -> Ts/2/1
  Sum1/1 -> inversion/1

== system simetranss/Machines/MATE Synchronous Machine/SSS-SM equations/Subsystem1 ==
  In1 : Inport
  Demux : Demux  Outputs=[5 1 ]
  Mux : Mux  Inputs=2
  u1 : Constant  Value=0
  Out1 : Outport
  wires:
  Mux/1 -> Out1/1
  Demux/1 -> Mux/1
  u1/1 -> Mux/2
  In1/1 -> Demux/1

== system simetranss/Machines/MATE Synchronous Machine/SSS-SM equations zero sequence only/Discretize ==
  Ac : Inport
  Bc : Inport  Port=2
  Unity : Inport  Port=3
  Product1 : Product  Multiplication=Matrix(*)  SaturateOnIntegerOverflow=on  OutDataTypeStr=Inherit: Same as first input
  Product4 : Product  Multiplication=Matrix(*)  SaturateOnIntegerOverflow=on  OutDataTypeStr=Inherit: Same as first input
  Sum1 : Sum  Inputs=+-  SaturateOnIntegerOverflow=on
  Sum5 : Sum  SaturateOnIntegerOverflow=on
  Ts/2 : Gain  Gain=Ts/2  SaturateOnIntegerOverflow=on  OutDataTypeStr=Inherit: Same as input  ParamDataTypeStr=Inherit: Same as input
  inversion : Product  Inputs=/  Multiplication=Matrix(*)  RndMeth=Zero
  trapeze has Ts/2 factor on B : Gain  Gain=Ts/2  SaturateOnIntegerOverflow=on  OutDataTypeStr=Inherit: Same as input  ParamDataTypeStr=Inherit: Same as input
  Ad : Outport
  Bd : Outport  Port=2
  wires:
  inversion/1 -> Product4/1, Product1/1  "inv(I4-Ts/2*A)"
  Bc/1 -> trapeze has Ts/2 factor on B/1
  trapeze has Ts/2 factor on B/1 -> Product1/2
  Ts/2/1 -> Sum5/2, Sum1/2
  Product4/1 -> Ad/1
  Unity/1 -> Sum5/1, Sum1/1
  Sum5/1 -> Product4/2
  Product1/1 -> Bd/1
  Ac/1 -> Ts/2/1
  Sum1/1 -> inversion/1

== system simetranss/Machines/MATE Synchronous Machine/Saturation/Lad ==
  note: Lad =1/(1/Lmd+1/Ll+1/Llkd+1/Llfd)
  Lmd : Inport
  Math Function2 : Math  Operator=reciprocal  SignedPower=on
  Math Function3 : Math  Operator=reciprocal  SignedPower=on
  Mux2 : Mux  Inputs=[3 1]
  Sum1 : Sum  Inputs=+  SaturateOnIntegerOverflow=on
  u1 : Constant  Value=[1/Lls 1/Llkd 1/Llf]
  Lad : Outport
  wires:
  Math Function2/1 -> Mux2/2
  Lmd/1 -> Math Function2/1
  Math Function3/1 -> Lad/1
  Sum1/1 -> Math Function3/1
  Mux2/1 -> Sum1/1
  u1/1 -> Mux2/1

== system simetranss/Machines/MATE Synchronous Machine/Saturation/Laq ==
  note: Laq = 1/(1/Lmq+1Ll+1/Llkq1+1/Llkq2)
  Lmq : Inport
  Math Function : Math  Operator=reciprocal  SignedPower=on
  Math Function1 : Math  Operator=reciprocal  SignedPower=on
  Mux1 : Mux  Inputs=[3 1]
  Sum2 : Sum  Inputs=+  SaturateOnIntegerOverflow=on
  u2 : Constant  Value=[ 1/Lls 1/Llkq 1/Llkq2]
  Laq : Outport
  wires:
  u2/1 -> Mux1/1
  Mux1/1 -> Sum2/1
  Sum2/1 -> Math Function1/1
  Math Function1/1 -> Laq/1
  Lmq/1 -> Math Function/1
  Math Function/1 -> Mux1/2

== system simetranss/Machines/MATE Synchronous Machine/Saturation/phimd ==
  note: phimd= phids*(Lad/Lls) +phifd*(Lad/Llfd) + phikd*(Lad/Llkd)
  phi : Inport
  Lad : Inport  Port=2
  1/Ll_d : Gain  Gain="[ 1/Lls   1/Llf   1/Llkd ]"  SaturateOnIntegerOverflow=on  OutDataTypeStr=Inherit: Same as input  ParamDataTypeStr=Inherit: Same as input
  Product4 : Product  RndMeth=Zero
  "phid phifd phikd " : Selector  InputPortWidth=7  IndexOptions=Index vector (dialog)  Indices=[1 3 4]  OutputSizes=1
  sum2 : Sum  Inputs=+  InputSameDT=on  SaturateOnIntegerOverflow=on  OutDataTypeStr=Inherit: Same as first input
  phimd : Outport
  wires:
  Lad/1 -> Product4/2
  Product4/1 -> phimd/1  "phimd"
  phi/1 -> "phid phifd phikd "/1
  1/Ll_d/1 -> sum2/1
  "phid phifd phikd "/1 -> 1/Ll_d/1
  sum2/1 -> Product4/1  "phimd"

== system simetranss/Machines/MATE Synchronous Machine/Saturation/phimq ==
  note: phimq= phiqs*(Laq/Lls) +phikq1*(Laq/Llkq1) +phikq2*(Laq/Llkq2)
  Laq : Inport
  phi : Inport  Port=2
  1/Ll_q : Gain  Gain=[1/Lls 1/Llkq 1/Llkq2]  SaturateOnIntegerOverflow=on  OutDataTypeStr=Inherit: Same as input  ParamDataTypeStr=Inherit: Same as input
  Product3 : Product  RndMeth=Zero
  phiq phikq1 (phikq2) : Selector  InputPortWidth=7  IndexOptions=Index vector (dialog)  Indices=[2 5 6]  OutputSizes=1
  sum1 : Sum  Inputs=+  InputSameDT=on  SaturateOnIntegerOverflow=on  OutDataTypeStr=Inherit: Same as first input
  phimq : Outport
  wires:
  phi/1 -> phiq phikq1 (phikq2)/1
  Product3/1 -> phimq/1  "phimq"
  Laq/1 -> Product3/2
  sum1/1 -> Product3/1  "phimq"
  phiq phikq1 (phikq2)/1 -> 1/Ll_q/1
  1/Ll_q/1 -> sum1/1

== system simetranss/Misc/Discrete Mean value/Model/Discrete Variable Time Delay ==
  In : Inport  SampleTime=Ts
  D : Inport  Port=2  SampleTime=Ts
  S-Function : S-Function  FunctionName=sfun_discreteVariableDelay  Parameters=MaxDelay,Ts,InitialValue,DFT  SFunctionDeploymentMode=off  EnableBusSupport=off
  Out : Outport  SampleTime=Ts  VectorParamsAs1DForOutWhenUnconnected=off
  wires:
  S-Function/1 -> Out/1
  In/1 -> S-Function/1
  D/1 -> S-Function/2
